simulink model "EngReq_SmkLimCalc"  (R2018a)
settings: configuration reference "cs_ert" (kept outside this file)
model workspace (MAT data in the model file):
  EngReq_SmkLimCalc_DT = 10
values from neighbouring files (symbols this model uses):
  EngReq_bSmkLimCnv_C = 0.0    [EngReq_SmkLimCalc.sldd]
  EngReq_bSmkLimIntkP_C = 0.0    [EngReq_SmkLimCalc.sldd]
  EngReq_facAFSFlt_C = 50.0    [EngReq_SmkLimCalc.sldd]
  EngReq_nSlpLimMin_C = 6000.0    [EngReq_SmkLimCalc.sldd]
  EngReq_SlpLimNeg_C = 50.0    [EngReq_SmkLimCalc.sldd]
  EngReq_SlpLimPos_C = 50.0    [EngReq_SmkLimCalc.sldd]
  SmkLim_facSmkATSCor_CUR : value not decoded    [EngReq_SmkLimCalc.sldd]
  SmkLim_facSmkATSCor_CURX : value not decoded    [EngReq_SmkLimCalc.sldd]
  SmkLim_facSmkEnvPCor_CUR : value not decoded    [EngReq_SmkLimCalc.sldd]
  SmkLim_facSmkEnvPCor_CURX : value not decoded    [EngReq_SmkLimCalc.sldd]
  SmkLim_trqLimSmk_MAP = 260.0 260.0 260.0 260.0 260.0 260.0 260.0 260.0 260.0 260.0 260.0 260.0 260.0 260.0 260.0 260.0 260.0 260.0 258.0078125 258.0078125 258.0078125 258.0078125 258.0078125 260.0 260.0 260.0 260.0 228.0078125 256.6015625 264.609375 276.015625 286.015625 295.9765625 299.9609375 299.9609375 299.9609375 195.7421875 194.296875 227.1484375 249.296875 252.5 271.7578125 286.875 298.59375 310.9375 191.3671875    [EngReq_SmkLimCalc.sldd]
  SmkLim_trqLimSmk_MAPX : value not decoded    [EngReq_SmkLimCalc.sldd]
  SmkLim_trqLimSmk_MAPY : value not decoded    [EngReq_SmkLimCalc.sldd]
  SmkLim_trqLimSmkAFS_MAP = 1000.0 1000.0 1000.0 1000.0 1000.0 1000.0 1000.0 1000.0 1000.0 1000.0 1000.0 1000.0 1000.0 1000.0 1000.0 1000.0 1000.0 1000.0 1000.0 1000.0 1000.0 1000.0 1000.0 1000.0 1000.0 1000.0 1000.0 1000.0 1000.0 1000.0 1000.0 1000.0 1000.0 1000.0 1000.0 1000.0 1000.0 1000.0 1000.0 1000.0 1000.0 1000.0 1000.0 1000.0 1000.0 1000.0 1000.0 1000.0 1000.0 1000.0 1000.0 1000.0 1000.0 1000.0 1000.0 1000.0 1000.0 1    [EngReq_SmkLimCalc.sldd]
  SmkLim_trqLimSmkAFS_MAPX : value not decoded    [EngReq_SmkLimCalc.sldd]
  SmkLim_trqLimSmkAFS_MAPY : value not decoded    [EngReq_SmkLimCalc.sldd]
  SmkLim_trqLimSmkAFSEnvPCor_MAP = 0.0 0.0 0.0 0.0 0.0 0.0 0.0 0.0 0.0 0.0 0.0 0.0 0.0 0.0 0.0 0.0 0.0 0.0 0.0 0.0 0.0 0.0 0.0 0.0 0.0 0.0 0.0 0.0 0.0 0.0 0.0 0.0 0.0 0.0 0.0 0.0 0.0 0.0 0.0 0.0 0.0 0.0 0.0 0.0 0.0 0.0 0.0 0.0 0.0 0.0 0.0 0.0 0.0 0.0 0.0 0.0 0.0 0.0 0.0 0.0 0.0 0.0 0.0 0.0 0.0 0.0 0.0 0.0 0.0 0.0 0.0 0.0 0.0 0.0 0.0 0.0 0.0 0.0 0.0 0.0 0.0 0.0 0.0 0.0 0.0 0.0 0.0 0.0 0.0 0.0 0.0 0.0 0.0 0.0 0.0 0.0 0.0 0.0 0.0 0.0    [EngReq_SmkLimCalc.sldd]
  SmkLim_trqLimSmkAFSEnvPCor_MAPX : value not decoded    [EngReq_SmkLimCalc.sldd]
  SmkLim_trqLimSmkAFSEnvPCor_MAPY : value not decoded    [EngReq_SmkLimCalc.sldd]
undefined symbols (not defined in the file or in its folder): CEngDsT_tTransf_CURX
libraries: sllib x2
settings Model: DataDictionary=EngReq_SmkLimCalc.sldd  Creator=zhoutinglin  LastModifiedBy=zhoutinglin

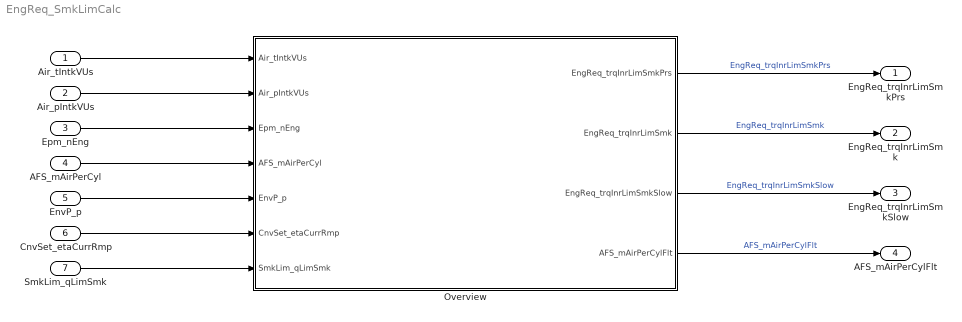
== system EngReq_SmkLimCalc ==
  Air_tIntkVUs : Inport  Description=Intake air temperature upstream of the inlet valve  OutMin=-200  OutMax=200  OutDataTypeStr=Temp_C  Unit=deg  PortDimensions=[1 1]
  Air_pIntkVUs : Inport  Description=Intake valve upstream pressure  Port=2  OutMin=0  OutMax=1200  OutDataTypeStr=Press_kpa  Unit=kPa  PortDimensions=[1 1]
  Epm_nEng : Inport  Description=Engine speed  Port=3  OutMin=0  OutMax=6000  OutDataTypeStr=ERPM  Unit=rpm  PortDimensions=[1 1]
  AFS_mAirPerCyl : Inport  Description=Air mass per cylinder  Port=4  OutMin=0  OutMax=16383  OutDataTypeStr=Mass_mg  Unit=mg/hub  PortDimensions=[1 1]
  EnvP_p : Inport  Description=Barometric pressure  Port=5  OutMin=0  OutMax=3276  OutDataTypeStr=Press_kpa  Unit=kPa  PortDimensions=[1 1]
  CnvSet_etaCurrRmp : Inport  Description=Conversion efficiency corresponding to CnvSet_qSet  Port=6  OutMin=-100  OutMax=100  OutDataTypeStr=Effcy  Unit=Nm/(mg/hub)  PortDimensions=[1 1]
  SmkLim_qLimSmk : Inport  Description=Smoke limitation quantity in current operation mode  Port=7  OutMin=-319  OutMax=319  OutDataTypeStr=InjMass  Unit=mg/hub  PortDimensions=[1 1]
  Overview : Subsystem
  EngReq_trqInrLimSmkPrs : Outport
  EngReq_trqInrLimSmk : Outport  Port=2
  EngReq_trqInrLimSmkSlow : Outport  Port=3
  AFS_mAirPerCylFlt : Outport  Port=4
  wires:
  Air_tIntkVUs/1 -> Overview/1(Air_tIntkVUs)
  Air_pIntkVUs/1 -> Overview/2(Air_pIntkVUs)
  Epm_nEng/1 -> Overview/3(Epm_nEng)
  AFS_mAirPerCyl/1 -> Overview/4(AFS_mAirPerCyl)
  EnvP_p/1 -> Overview/5(EnvP_p)
  CnvSet_etaCurrRmp/1 -> Overview/6(CnvSet_etaCurrRmp)
  SmkLim_qLimSmk/1 -> Overview/7(SmkLim_qLimSmk)
  Overview/1(EngReq_trqInrLimSmkPrs) -> EngReq_trqInrLimSmkPrs/1  "EngReq_trqInrLimSmkPrs"
  Overview/2(EngReq_trqInrLimSmk) -> EngReq_trqInrLimSmk/1  "EngReq_trqInrLimSmk"
  Overview/3(EngReq_trqInrLimSmkSlow) -> EngReq_trqInrLimSmkSlow/1  "EngReq_trqInrLimSmkSlow"
  Overview/4(AFS_mAirPerCylFlt) -> AFS_mAirPerCylFlt/1  "AFS_mAirPerCylFlt"

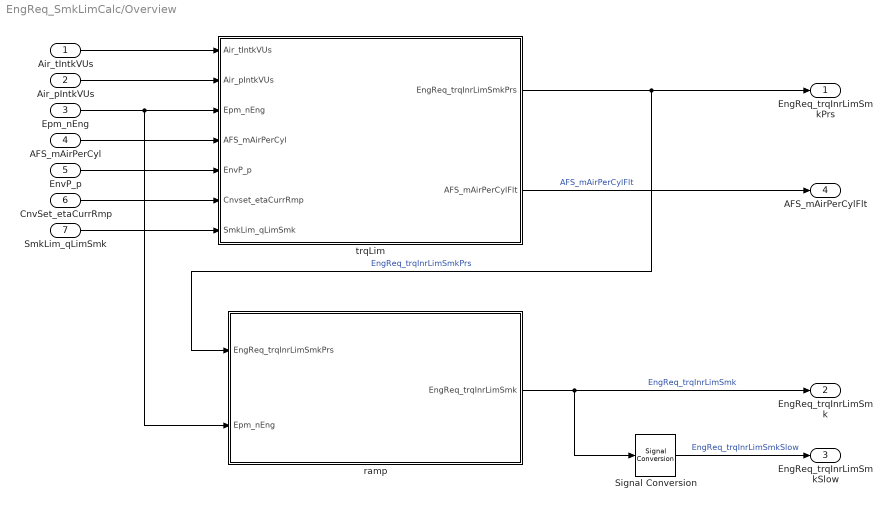
== system EngReq_SmkLimCalc/Overview ==
  Air_tIntkVUs : Inport  Tag=deg
  Air_pIntkVUs : Inport  Tag=kPa  Port=2
  Epm_nEng : Inport  Tag=rpm  Port=3
  AFS_mAirPerCyl : Inport  Tag=mg/hub  Port=4
  EnvP_p : Inport  Tag=kPa  Port=5
  CnvSet_etaCurrRmp : Inport  Tag=Nm/(mg/hub)  Port=6
  SmkLim_qLimSmk : Inport  Tag=mg/hub  Port=7
  Signal Conversion : SignalConversion  OverrideOpt=off
  ramp : Subsystem
  trqLim : Subsystem
  EngReq_trqInrLimSmkPrs : Outport  Tag=Nm
  EngReq_trqInrLimSmk : Outport  Tag=Nm  Port=2
  EngReq_trqInrLimSmkSlow : Outport  Tag=Nm  Port=3
  AFS_mAirPerCylFlt : Outport  Tag=mg/hub  Port=4
  wires:
  Air_tIntkVUs/1 -> trqLim/1(Air_tIntkVUs)
  trqLim/2(AFS_mAirPerCylFlt) -> AFS_mAirPerCylFlt/1  "AFS_mAirPerCylFlt"
  Air_pIntkVUs/1 -> trqLim/2(Air_pIntkVUs)
  EnvP_p/1 -> trqLim/5(EnvP_p)
  SmkLim_qLimSmk/1 -> trqLim/7(SmkLim_qLimSmk)
  trqLim/1(EngReq_trqInrLimSmkPrs) -> ramp/1(EngReq_trqInrLimSmkPrs), EngReq_trqInrLimSmkPrs/1  "EngReq_trqInrLimSmkPrs"
  Signal Conversion/1 -> EngReq_trqInrLimSmkSlow/1  "EngReq_trqInrLimSmkSlow"
  AFS_mAirPerCyl/1 -> trqLim/4(AFS_mAirPerCyl)
  CnvSet_etaCurrRmp/1 -> trqLim/6(Cnvset_etaCurrRmp)
  ramp/1(EngReq_trqInrLimSmk) -> Signal Conversion/1, EngReq_trqInrLimSmk/1  "EngReq_trqInrLimSmk"
  Epm_nEng/1 -> ramp/2(Epm_nEng), trqLim/3(Epm_nEng)

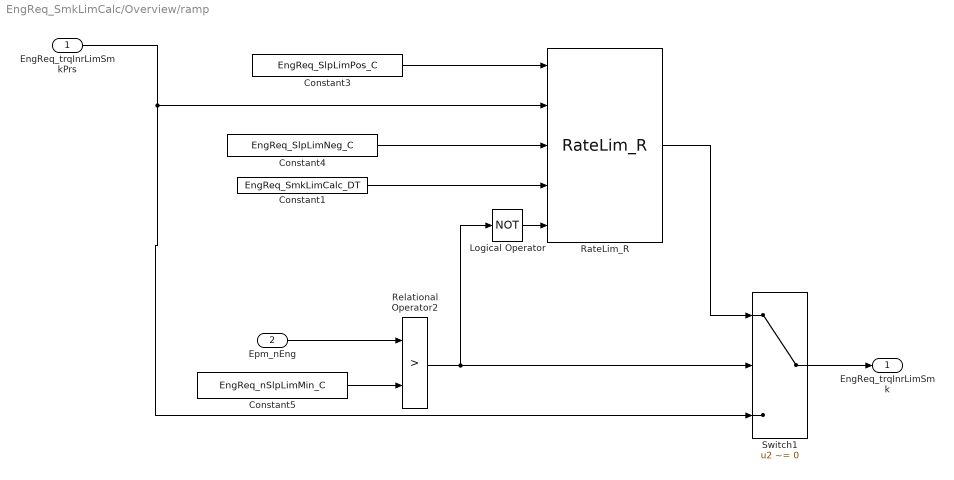
== system EngReq_SmkLimCalc/Overview/ramp ==
  EngReq_trqInrLimSmkPrs : Inport
  Epm_nEng : Inport  Port=2
  Constant1 : Constant  Value=EngReq_SmkLimCalc_DT
  Constant3 : Constant  Value=EngReq_SlpLimPos_C
  Constant4 : Constant  Value=EngReq_SlpLimNeg_C
  Constant5 : Constant  Value=EngReq_nSlpLimMin_C
  Logical Operator : Logic  Operator=NOT  AllPortsSameDT=off  OutDataTypeStr=boolean
  RateLim_R : sllib/RateLim_R
      settings: SourceProductName=sllib
  Relational Operator2 : RelationalOperator  Operator=>  OutDataTypeStr=boolean  RndMeth=Nearest  InputSameDT=on
  Switch1 : Switch  Criteria=u2 ~= 0  SaturateOnIntegerOverflow=on  InputSameDT=on
  EngReq_trqInrLimSmk : Outport
  wires:
  Epm_nEng/1 -> Relational Operator2/1
  Switch1/1 -> EngReq_trqInrLimSmk/1
  Constant1/1 -> RateLim_R/4
  Constant4/1 -> RateLim_R/3
  RateLim_R/1 -> Switch1/1
  Constant3/1 -> RateLim_R/1
  Constant5/1 -> Relational Operator2/2
  Logical Operator/1 -> RateLim_R/5
  Relational Operator2/1 -> Switch1/2, Logical Operator/1
  EngReq_trqInrLimSmkPrs/1 -> RateLim_R/2, Switch1/3

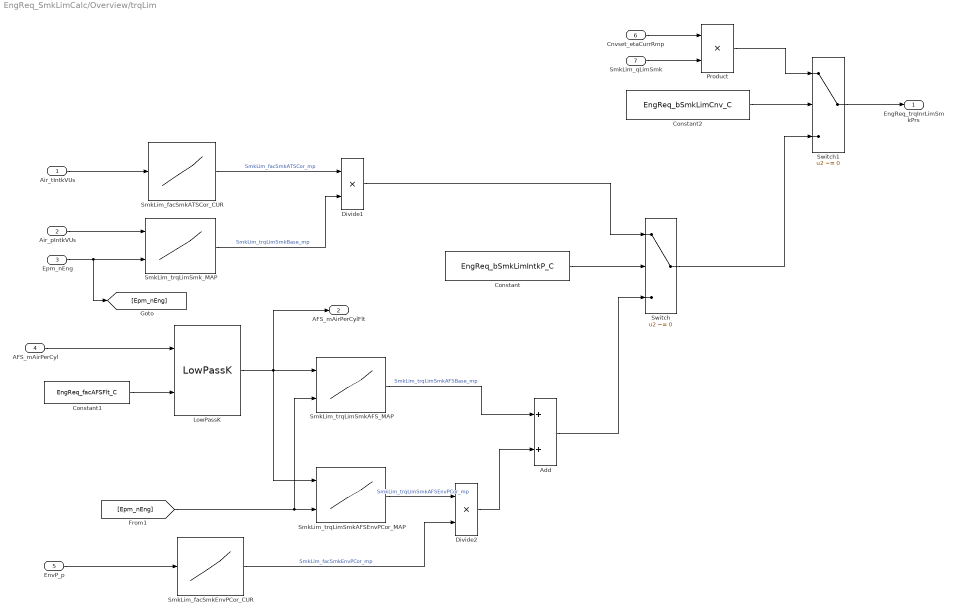
== system EngReq_SmkLimCalc/Overview/trqLim ==
  Air_tIntkVUs : Inport
  Air_pIntkVUs : Inport  Port=2
  Epm_nEng : Inport  Port=3
  AFS_mAirPerCyl : Inport  Port=4
  EnvP_p : Inport  Port=5
  Cnvset_etaCurrRmp : Inport  Tag=Nm/(mg/hub)  Port=6
  SmkLim_qLimSmk : Inport  Tag=mg/hub  Port=7
  Add : Sum  SaturateOnIntegerOverflow=on  InputSameDT=on  OutDataTypeStr=Inherit: Same as first input
  Constant : Constant  Value=EngReq_bSmkLimIntkP_C
  Constant1 : Constant  Value=EngReq_facAFSFlt_C
  Constant2 : Constant  Value=EngReq_bSmkLimCnv_C
  Divide1 : Product  Inputs=**  OutDataTypeStr=Inherit: Inherit via back propagation  RndMeth=Round  SaturateOnIntegerOverflow=on
  Divide2 : Product  Inputs=**  OutDataTypeStr=Inherit: Inherit via back propagation  RndMeth=Round  SaturateOnIntegerOverflow=on
  LowPassK : sllib/LowPassK
      settings: SourceProductName=sllib
  Product : Product  OutDataTypeStr=Inherit: Inherit via back propagation  SaturateOnIntegerOverflow=on
  SmkLim_facSmkATSCor_CUR : Lookup_n-D  DialogController=Simulink.DDGSource  NumberOfTableDimensions=1  BreakpointsForDimension1=SmkLim_facSmkATSCor_CURX  BreakpointsForDimension2=CEngDsT_tTransf_CURX  IndexSearchMethod=Linear search  BeginIndexSearchUsingPreviousIndexResult=on  Table=SmkLim_facSmkATSCor_CUR  ExtrapMethod=Clip  UseLastTableValue=on  InternalRulePriority=Speed  OutDataTypeStr=Inherit: Inherit via back propagation  SaturateOnIntegerOverflow=on
  SmkLim_facSmkEnvPCor_CUR : Lookup_n-D  DialogController=Simulink.DDGSource  NumberOfTableDimensions=1  BreakpointsForDimension1=SmkLim_facSmkEnvPCor_CURX  BreakpointsForDimension2=CEngDsT_tTransf_CURX  BreakpointsForDimension1DataTypeStr=Inherit: Inherit from 'Breakpoint data'  IndexSearchMethod=Linear search  BeginIndexSearchUsingPreviousIndexResult=on  Table=SmkLim_facSmkEnvPCor_CUR  TableDataTypeStr=Inherit: Inherit from 'Table data'  ExtrapMethod=Clip  UseLastTableValue=on  InternalRulePriority=Speed  OutDataTypeStr=Inherit: Inherit from 'Table data'  SaturateOnIntegerOverflow=on
  SmkLim_trqLimSmkAFSEnvPCor_MAP : Lookup_n-D  BreakpointsForDimension1=SmkLim_trqLimSmkAFSEnvPCor_MAPY  BreakpointsForDimension2=SmkLim_trqLimSmkAFSEnvPCor_MAPX  IndexSearchMethod=Linear search  BeginIndexSearchUsingPreviousIndexResult=on  Table=SmkLim_trqLimSmkAFSEnvPCor_MAP  ExtrapMethod=Clip  UseLastTableValue=on  InternalRulePriority=Speed  OutDataTypeStr=Inherit: Inherit via back propagation  RndMeth=Simplest  SaturateOnIntegerOverflow=on
  SmkLim_trqLimSmkAFS_MAP : Lookup_n-D  BreakpointsForDimension1=SmkLim_trqLimSmkAFS_MAPY  BreakpointsForDimension2=SmkLim_trqLimSmkAFS_MAPX  IndexSearchMethod=Linear search  BeginIndexSearchUsingPreviousIndexResult=on  Table=SmkLim_trqLimSmkAFS_MAP  ExtrapMethod=Clip  UseLastTableValue=on  InternalRulePriority=Speed  OutDataTypeStr=Inherit: Inherit via back propagation  RndMeth=Simplest  SaturateOnIntegerOverflow=on
  SmkLim_trqLimSmk_MAP : Lookup_n-D  BreakpointsForDimension1=SmkLim_trqLimSmk_MAPY  BreakpointsForDimension2=SmkLim_trqLimSmk_MAPX  IndexSearchMethod=Linear search  BeginIndexSearchUsingPreviousIndexResult=on  Table=SmkLim_trqLimSmk_MAP  ExtrapMethod=Clip  UseLastTableValue=on  InternalRulePriority=Speed  OutDataTypeStr=Inherit: Inherit via back propagation  RndMeth=Simplest  SaturateOnIntegerOverflow=on
  Switch : Switch  Criteria=u2 ~= 0  InputSameDT=on
  Switch1 : Switch  Criteria=u2 ~= 0  InputSameDT=on
  EngReq_trqInrLimSmkPrs : Outport
  AFS_mAirPerCylFlt : Outport  Tag=mg/hub  Port=2
  wires:
  [Epm_nEng] -> SmkLim_trqLimSmkAFS_MAP/2, SmkLim_trqLimSmkAFSEnvPCor_MAP/2
  Epm_nEng/1 -> [Epm_nEng], SmkLim_trqLimSmk_MAP/2
  SmkLim_trqLimSmk_MAP/1 -> Divide1/2  "SmkLim_trqLimSmkBase_mp"
  Air_tIntkVUs/1 -> SmkLim_facSmkATSCor_CUR/1
  Air_pIntkVUs/1 -> SmkLim_trqLimSmk_MAP/1
  SmkLim_facSmkATSCor_CUR/1 -> Divide1/1  "SmkLim_facSmkATSCor_mp"
  LowPassK/1 -> AFS_mAirPerCylFlt/1, SmkLim_trqLimSmkAFSEnvPCor_MAP/1, SmkLim_trqLimSmkAFS_MAP/1
  AFS_mAirPerCyl/1 -> LowPassK/1
  Add/1 -> Switch/3
  Divide1/1 -> Switch/1
  SmkLim_trqLimSmkAFS_MAP/1 -> Add/1  "SmkLim_trqLimSmkAFSBase_mp"
  SmkLim_trqLimSmkAFSEnvPCor_MAP/1 -> Divide2/1  "SmkLim_trqLimSmkAFSEnvPCor_mp"
  EnvP_p/1 -> SmkLim_facSmkEnvPCor_CUR/1
  SmkLim_facSmkEnvPCor_CUR/1 -> Divide2/2  "SmkLim_facSmkEnvPCor_mp"
  Divide2/1 -> Add/2
  Constant/1 -> Switch/2
  Switch1/1 -> EngReq_trqInrLimSmkPrs/1
  Switch/1 -> Switch1/3
  Constant2/1 -> Switch1/2
  Cnvset_etaCurrRmp/1 -> Product/1
  SmkLim_qLimSmk/1 -> Product/2
  Product/1 -> Switch1/1
  Constant1/1 -> LowPassK/2
